simulink model "sl_subsys_fcncallerr15"  (Simulink 7.6)
settings: Solver=FixedStepDiscrete  StartTime=0.0  StopTime=10.0  RelTol=1e-3
libraries: simulink x2
settings Model: Creator=The MathWorks Inc.
settings DataIOCC: SaveState=on
settings DebuggingCC: UnderspecifiedInitializationDetection=Simplified  StrictBusMsg=ErrorOnBusTreatedAsVector
settings SFSimCC: SimParseCustomCode=off

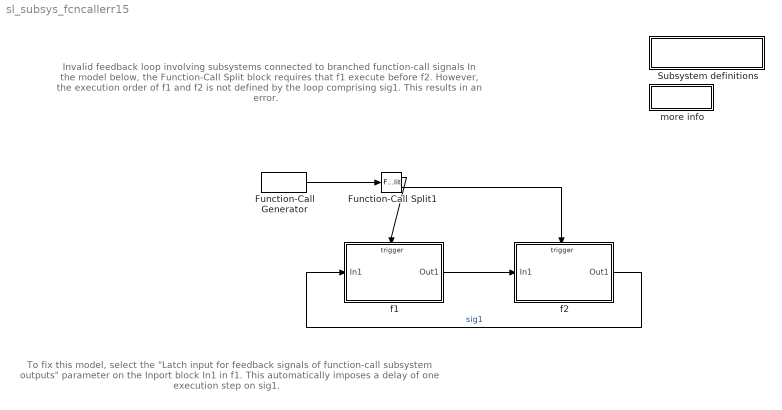
== system sl_subsys_fcncallerr15 ==
  note: Invalid feedback loop involving subsystems connected to branched
      | function-call signals
      |
      | In the model below, the Function-Call Split block requires that f1 execute
      | before f2. However, the execution order of f1 and f2 is not defined by the
      | loop comprising sig1. This results in an error.
  note: To fix this model, select the "Latch input for feedback signals of function-call
      | subsystem outputs" parameter on the Inport block In1 in f1. This automatically
      | imposes a delay of one execution step on sig1.
  " Subsystem definitions" : Subsystem
      settings: OpenFcn=helpview([matlabroot,'/toolbox/simulink/simdemos/simfeatures/html/sl_subsys_definitions.html']);
      mask Display: disp('Subsystem\ndefinitions')
  Function-Call Generator : simulink/Ports & Subsystems/Function-Call Generator  sample_time=1  numberOfIterations=1
  Function-Call Split1 : FunctionCallSplit
  f1 : Subsystem  TreatAsAtomicUnit=on
  f2 : Subsystem  TreatAsAtomicUnit=on
  more info : Subsystem
      mask Display: disp(get_param(gcb,'name'))
  wires:
  Function-Call Generator/1 -> Function-Call Split1/1
  f2/1(Out1) -> f1/1(In1)  "sig1"
  Function-Call Split1/1 -> f1/Trigger
  Function-Call Split1/2 -> f2/Trigger
  f1/1(Out1) -> f2/1(In1)

== system sl_subsys_fcncallerr15/ Subsystem definitions ==

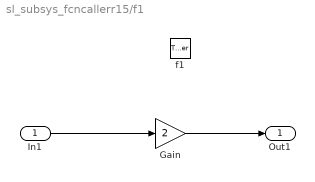
== system sl_subsys_fcncallerr15/f1 ==
  In1 : Inport
  f1 : TriggerPort  TriggerType=function-call  SampleTimeType=periodic
  Gain : Gain  Gain=2
  Out1 : Outport  InitialOutput=1/1000
      settings: AttributesFormatString=%<OutputWhenDisabled>: %<InitialOutput>
  wires:
  Gain/1 -> Out1/1
  In1/1 -> Gain/1

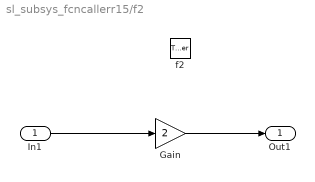
== system sl_subsys_fcncallerr15/f2 ==
  In1 : Inport
  f2 : TriggerPort  TriggerType=function-call  SampleTimeType=periodic
  Gain : Gain  Gain=2
  Out1 : Outport  InitialOutput=1/1000
      settings: AttributesFormatString=%<OutputWhenDisabled>: %<InitialOutput>
  wires:
  In1/1 -> Gain/1
  Gain/1 -> Out1/1

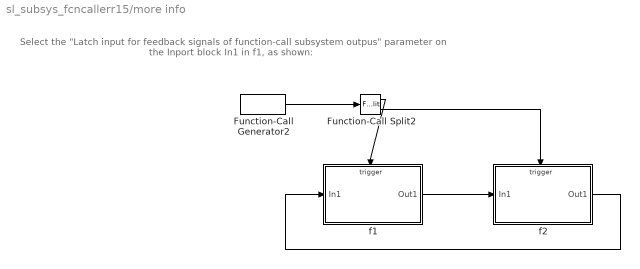
== system sl_subsys_fcncallerr15/more info ==
  note: Select the "Latch input for feedback signals of function-call subsystem outpus"
      | parameter on the Inport block In1 in f1, as shown:
  Function-Call Generator2 : simulink/Ports & Subsystems/Function-Call Generator  sample_time=1  numberOfIterations=1
  Function-Call Split2 : FunctionCallSplit
  f1 : Subsystem  TreatAsAtomicUnit=on
  f2 : Subsystem  TreatAsAtomicUnit=on
  wires:
  f2/1(Out1) -> f1/1(In1)
  Function-Call Split2/1 -> f1/Trigger
  Function-Call Split2/2 -> f2/Trigger
  f1/1(Out1) -> f2/1(In1)
  Function-Call Generator2/1 -> Function-Call Split2/1

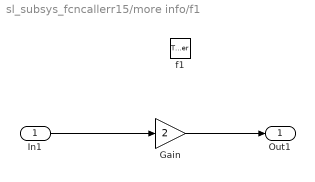
== system sl_subsys_fcncallerr15/more info/f1 ==
  In1 : Inport
      settings: LatchInputForFeedbackSignals=on
  f1 : TriggerPort  TriggerType=function-call  SampleTimeType=periodic
  Gain : Gain  Gain=2
  Out1 : Outport  InitialOutput=1/1000
      settings: AttributesFormatString=%<OutputWhenDisabled>: %<InitialOutput>
  wires:
  In1/1 -> Gain/1
  Gain/1 -> Out1/1

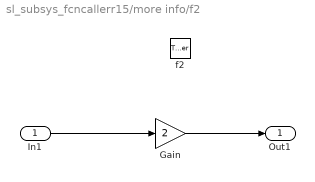
== system sl_subsys_fcncallerr15/more info/f2 ==
  In1 : Inport
  f2 : TriggerPort  TriggerType=function-call  SampleTimeType=periodic
  Gain : Gain  Gain=2
  Out1 : Outport  InitialOutput=1/1000
      settings: AttributesFormatString=%<OutputWhenDisabled>: %<InitialOutput>
  wires:
  Gain/1 -> Out1/1
  In1/1 -> Gain/1
